simulink model "third"  (R2019b)
settings: Solver=VariableStepAuto  StartTime=0.0  StopTime=10.0  RelTol=1e-3
libraries: simulink x1
settings Model: Creator=Pranshu  LastModifiedBy=Pranshu

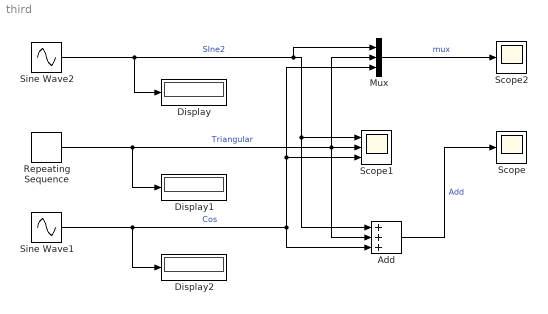
== system third ==
  Add : Sum  Inputs=+++
  Display : Display
  Display1 : Display
  Display2 : Display
  Mux : Mux  Inputs=3
  Repeating Sequence : simulink/Sources/Repeating Sequence  rep_seq_t=[0 2]  rep_seq_y=[0 5]
  Scope : Scope
  Scope1 : Scope  NumInputPorts=3
  Scope2 : Scope
  Sine Wave1 : Sin  Amplitude=2  Frequency=2  Phase=1.5707  SampleTime=0
  Sine Wave2 : Sin  Amplitude=3  Frequency=2  SampleTime=0
  wires:
  Repeating Sequence/1 -> Display1/1, Mux/2, Add/2, Scope1/2  "Triangular"
  Sine Wave2/1 -> Display/1, Mux/1, Add/1, Scope1/1  "SIne2"
  Sine Wave1/1 -> Display2/1, Mux/3, Scope1/3, Add/3  "Cos"
  Add/1 -> Scope/1  "Add"
  Mux/1 -> Scope2/1  "mux"
